simulink model "testing_model"  (R2024a)
settings: Solver=FixedStepAuto  StartTime=0.0  StopTime=60  FixedStep=Ts  RelTol=1e-3
values from neighbouring files (symbols this model uses):
  telescope0 = 0    [enviroment_setup.m]
  thetaList0 = [0, 0,-pi/8, 0, 0]'    [enviroment_setup.m]
  Ts = 0.001    [enviroment_setup.m]
libraries: TcSimInterface x2, sldrtlib x1
(part 2 of 2)

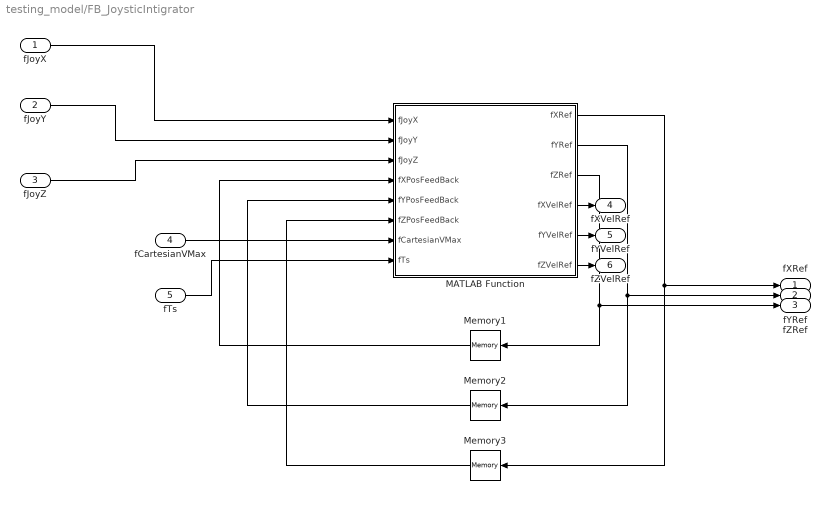
== system testing_model/FB_JoysticIntigrator ==
  fJoyX : Inport
  fJoyY : Inport  Port=2
  fJoyZ : Inport  Port=3
  fCartesianVMax : Inport  Port=4
  fTs : Inport  Port=5
  MATLAB Function : MATLAB Function  TreatAsAtomicUnit=on
  Memory1 : Memory
  Memory2 : Memory
  Memory3 : Memory
  fXRef : Outport
  fYRef : Outport  Port=2
  fZRef : Outport  Port=3
  fXVelRef : Outport  Port=4
  fYVelRef : Outport  Port=5
  fZVelRef : Outport  Port=6
  wires:
  Memory2/1 -> MATLAB Function/5(fYPosFeedBack)
  fJoyY/1 -> MATLAB Function/2(fJoyY)
  MATLAB Function/1(fXRef) -> fXRef/1, Memory3/1
  Memory1/1 -> MATLAB Function/4(fXPosFeedBack)
  MATLAB Function/2(fYRef) -> fYRef/1, Memory2/1
  fCartesianVMax/1 -> MATLAB Function/7(fCartesianVMax)
  Memory3/1 -> MATLAB Function/6(fZPosFeedBack)
  MATLAB Function/3(fZRef) -> fZRef/1, Memory1/1
  MATLAB Function/6(fZVelRef) -> fZVelRef/1
  MATLAB Function/4(fXVelRef) -> fXVelRef/1
  MATLAB Function/5(fYVelRef) -> fYVelRef/1
  fTs/1 -> MATLAB Function/8(fTs)
  fJoyX/1 -> MATLAB Function/1(fJoyX)
  fJoyZ/1 -> MATLAB Function/3(fJoyZ)

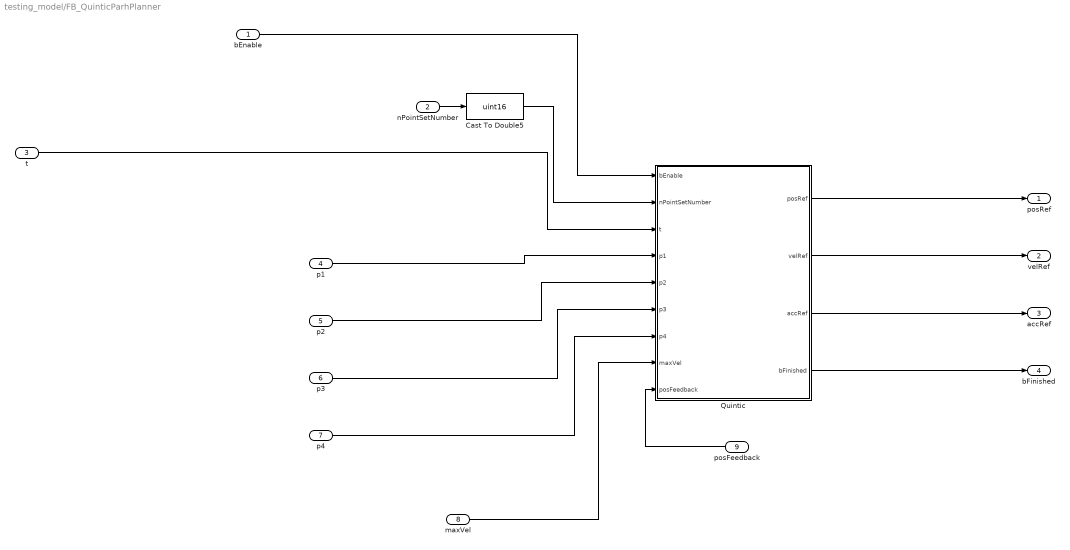
== system testing_model/FB_QuinticParhPlanner ==
  bEnable : Inport
  nPointSetNumber : Inport  Port=2
  t : Inport  Port=3
  p1 : Inport  Port=4
  p2 : Inport  Port=5
  p3 : Inport  Port=6
  p4 : Inport  Port=7
  maxVel : Inport  Port=8
  posFeedback : Inport  Port=9
  Cast To Double5 : DataTypeConversion  OutDataTypeStr=uint16  SaturateOnIntegerOverflow=off  RndMeth=Floor
  Quintic : MATLAB Function  TreatAsAtomicUnit=on
  posRef : Outport
  velRef : Outport  Port=2
  accRef : Outport  Port=3
  bFinished : Outport  Port=4
  wires:
  t/1 -> Quintic/3(t)
  p2/1 -> Quintic/5(p2)
  bEnable/1 -> Quintic/1(bEnable)
  maxVel/1 -> Quintic/8(maxVel)
  Quintic/4(bFinished) -> bFinished/1
  Quintic/2(velRef) -> velRef/1
  Quintic/1(posRef) -> posRef/1
  Quintic/3(accRef) -> accRef/1
  p1/1 -> Quintic/4(p1)
  p3/1 -> Quintic/6(p3)
  p4/1 -> Quintic/7(p4)
  posFeedback/1 -> Quintic/9(posFeedback)
  nPointSetNumber/1 -> Cast To Double5/1
  Cast To Double5/1 -> Quintic/2(nPointSetNumber)

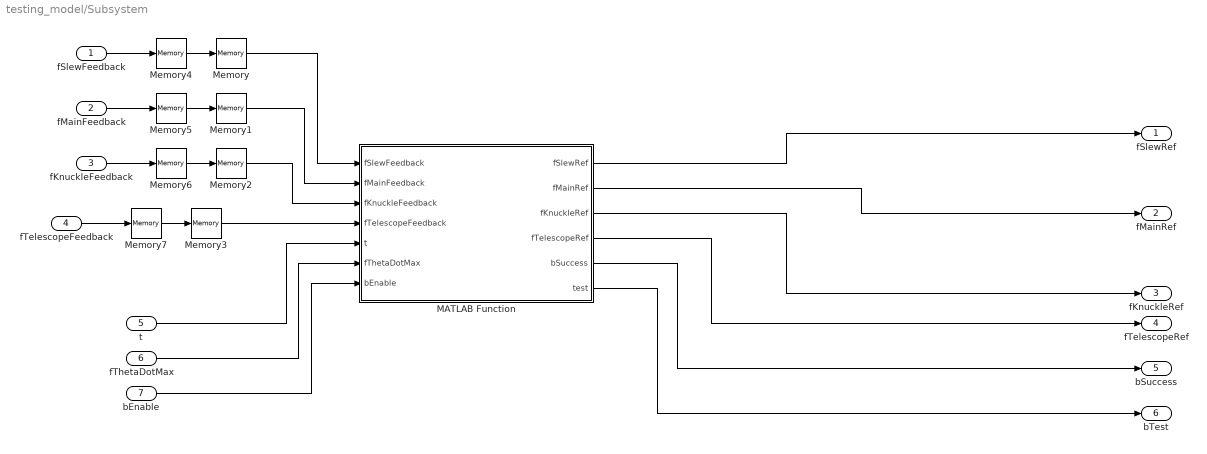
== system testing_model/Subsystem ==
  fSlewFeedback : Inport
  fMainFeedback : Inport  Port=2
  fKnuckleFeedback : Inport  Port=3
  fTelescopeFeedback : Inport  Port=4
  t : Inport  Port=5
  fThetaDotMax : Inport  Port=6
  bEnable : Inport  Port=7
  MATLAB Function : MATLAB Function  TreatAsAtomicUnit=on
  Memory : Memory  InitialCondition=thetaList0(1)
  Memory1 : Memory  InitialCondition=thetaList0(2)
  Memory2 : Memory  InitialCondition=thetaList0(3)
  Memory3 : Memory  InitialCondition=telescope0
  Memory4 : Memory  InitialCondition=thetaList0(1)
  Memory5 : Memory  InitialCondition=thetaList0(2)
  Memory6 : Memory  InitialCondition=thetaList0(3)
  Memory7 : Memory  InitialCondition=telescope0
  fSlewRef : Outport
  fMainRef : Outport  Port=2
  fKnuckleRef : Outport  Port=3
  fTelescopeRef : Outport  Port=4
  bSuccess : Outport  Port=5
  bTest : Outport  Port=6
  wires:
  MATLAB Function/4(fTelescopeRef) -> fTelescopeRef/1
  MATLAB Function/2(fMainRef) -> fMainRef/1
  fMainFeedback/1 -> Memory5/1
  fSlewFeedback/1 -> Memory4/1
  fKnuckleFeedback/1 -> Memory6/1
  MATLAB Function/5(bSuccess) -> bSuccess/1
  t/1 -> MATLAB Function/5(t)
  MATLAB Function/1(fSlewRef) -> fSlewRef/1
  MATLAB Function/3(fKnuckleRef) -> fKnuckleRef/1
  fThetaDotMax/1 -> MATLAB Function/6(fThetaDotMax)
  bEnable/1 -> MATLAB Function/7(bEnable)
  fTelescopeFeedback/1 -> Memory7/1
  Memory/1 -> MATLAB Function/1(fSlewFeedback)
  Memory1/1 -> MATLAB Function/2(fMainFeedback)
  Memory2/1 -> MATLAB Function/3(fKnuckleFeedback)
  Memory3/1 -> MATLAB Function/4(fTelescopeFeedback)
  Memory7/1 -> Memory3/1
  Memory4/1 -> Memory/1
  Memory5/1 -> Memory1/1
  Memory6/1 -> Memory2/1
  MATLAB Function/6(test) -> bTest/1

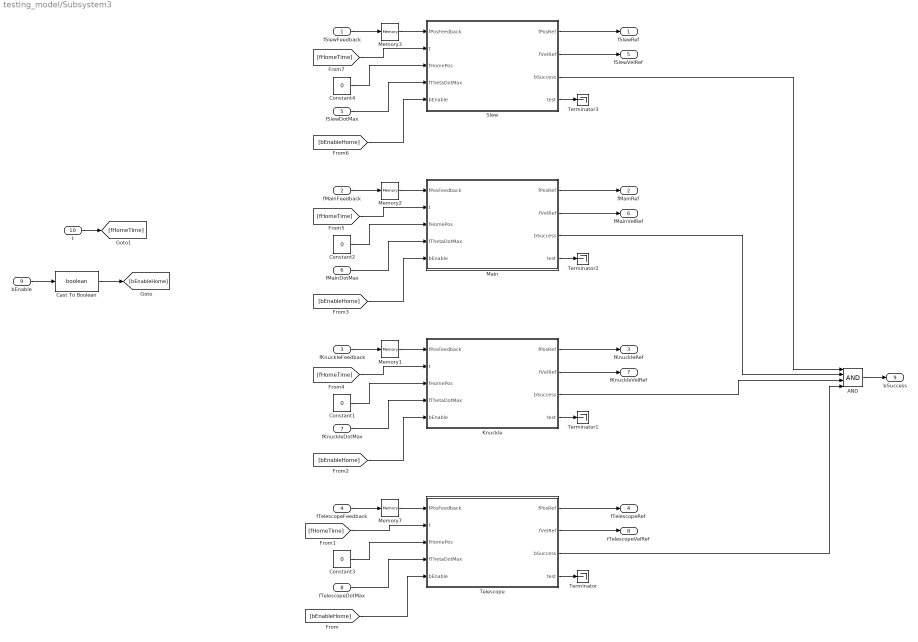
== system testing_model/Subsystem3 ==
  fSlewFeedback : Inport
  fMainFeedback : Inport  Port=2
  fKnuckleFeedback : Inport  Port=3
  fTelescopeFeedback : Inport  Port=4
  fSlewDotMax : Inport  Port=5
  fMainDotMax : Inport  Port=6
  fKnuckleDotMax : Inport  Port=7
  fTelescopeDotMax : Inport  Port=8
  bEnable : Inport  Port=9
  t : Inport  Port=10
  AND : Logic  Inputs=4  IconShape=distinctive  AllPortsSameDT=off  OutDataTypeStr=boolean
  Cast To Boolean : DataTypeConversion  OutDataTypeStr=boolean  SaturateOnIntegerOverflow=off  RndMeth=Floor
  Constant{1..4} (4 alike) : Constant  Value=0
  Knuckle : MATLAB Function  TreatAsAtomicUnit=on
  Main : MATLAB Function  TreatAsAtomicUnit=on
  Memory1 : Memory  InitialCondition=thetaList0(3)
  Memory2 : Memory  InitialCondition=thetaList0(2)
  Memory3 : Memory  InitialCondition=thetaList0(2)
  Memory7 : Memory  InitialCondition=telescope0
  Slew : MATLAB Function  TreatAsAtomicUnit=on
  Telescope : MATLAB Function  TreatAsAtomicUnit=on
  Terminator{,1..3} (4 alike) : Terminator
  fSlewRef : Outport
  fMainRef : Outport  Port=2
  fKnuckleRef : Outport  Port=3
  fTelescopeRef : Outport  Port=4
  fSlewVelRef : Outport  Port=5
  fMainVelRef : Outport  Port=6
  fKnuckleVelRef : Outport  Port=7
  fTelescopeVelRef : Outport  Port=8
  bSuccess : Outport  Port=9
  wires:
  Telescope/1(fPosRef) -> fTelescopeRef/1
  Telescope/3(bSuccess) -> AND/4
  [fHomeTime] -> Telescope/2(t)
  fTelescopeDotMax/1 -> Telescope/4(fThetaDotMax)
  [bEnableHome] -> Telescope/5(bEnable)
  fTelescopeFeedback/1 -> Memory7/1
  Constant3/1 -> Telescope/3(fHomePos)
  Memory7/1 -> Telescope/1(fPosFeedback)
  Telescope/2(fVelRef) -> fTelescopeVelRef/1
  Telescope/4(test) -> Terminator/1
  Constant1/1 -> Knuckle/3(fHomePos)
  Knuckle/3(bSuccess) -> AND/3
  Knuckle/2(fVelRef) -> fKnuckleVelRef/1
  Memory1/1 -> Knuckle/1(fPosFeedback)
  Knuckle/4(test) -> Terminator1/1
  Knuckle/1(fPosRef) -> fKnuckleRef/1
  [bEnableHome] -> Knuckle/5(bEnable)
  fKnuckleDotMax/1 -> Knuckle/4(fThetaDotMax)
  [fHomeTime] -> Knuckle/2(t)
  fKnuckleFeedback/1 -> Memory1/1
  AND/1 -> bSuccess/1
  bEnable/1 -> Cast To Boolean/1
  t/1 -> [fHomeTime]
  Cast To Boolean/1 -> [bEnableHome]
  Main/3(bSuccess) -> AND/2
  fMainDotMax/1 -> Main/4(fThetaDotMax)
  Main/4(test) -> Terminator2/1
  fMainFeedback/1 -> Memory2/1
  Memory2/1 -> Main/1(fPosFeedback)
  Main/2(fVelRef) -> fMainVelRef/1
  [bEnableHome] -> Main/5(bEnable)
  Constant2/1 -> Main/3(fHomePos)
  Main/1(fPosRef) -> fMainRef/1
  [fHomeTime] -> Main/2(t)
  [bEnableHome] -> Slew/5(bEnable)
  Slew/2(fVelRef) -> fSlewVelRef/1
  Memory3/1 -> Slew/1(fPosFeedback)
  Slew/3(bSuccess) -> AND/1
  Slew/4(test) -> Terminator3/1
  [fHomeTime] -> Slew/2(t)
  Slew/1(fPosRef) -> fSlewRef/1
  fSlewFeedback/1 -> Memory3/1
  Constant4/1 -> Slew/3(fHomePos)
  fSlewDotMax/1 -> Slew/4(fThetaDotMax)

== matlab function testing_model/FB_JoysticIntigrator/MATLAB Function ==
  data: fJoyX input; fJoyY input; fJoyZ input; fXPosFeedBack input; fXRef output; fYRef output; fZRef output; fXVelRef output; fYVelRef output; fZVelRef output; fYPosFeedBack input; fZPosFeedBack input; fCartesianVMax input; fTs input
function [fXRef, fYRef, fZRef, fXVelRef, fYVelRef, fZVelRef]  = fcn(fJoyX, fJoyY, fJoyZ, fXPosFeedBack, fYPosFeedBack, fZPosFeedBack, fCartesianVMax, fTs)

fXVelRef = fCartesianVMax*fJoyX;
fYVelRef = fCartesianVMax*fJoyY;
fZVelRef = fCartesianVMax*fJoyZ;

fXRef = fXPosFeedBack + fXVelRef*fTs;
fYRef = fYPosFeedBack + fYVelRef*fTs; 
fZRef = fZPosFeedBack + fZVelRef*fTs;

== matlab function testing_model/MATLAB Function3 ==
  settings: updateMethod=DISCRETE
  data: p1 input; p2 input; p3 input; xyzOut output; xyzDotOut output; t_current input; bEnable input; MaxVel input; pointSetNumber input; pointSetFromMemory input; pointSetToMemory output; xyzFeedback input; xyzDotFeedback input; tFromMemory input; tToMemory output
function [xyzOut, xyzDotOut, pointSetToMemory, tToMemory] = CubicPlanner(p1, p2, p3, t_current, bEnable, MaxVel, pointSetNumber, pointSetFromMemory, xyzFeedback, xyzDotFeedback,tFromMemory)
xyzOut = zeros(3, 1);
xyzDotOut = zeros(3, 1);
bFirstCycle = false;
bNewPointSet = false;


persistent tToSubtract;
if isempty(tToSubtract)
    tToSubtract = 0.0;
end

persistent bEnableMemory;
if isempty(bEnableMemory)
    bEnableMemory = false;
end

persistent p1Memory;
if isempty(p1Memory)
    p1Memory = p1;
end
persistent p2Memory;
if isempty(p2Memory)
    p2Memory = p2;
end
persistent p3Memory;
if isempty(p3Memory)
    p3Memory = p3;
end


% Detect first cykle
if (bEnable == true) && (bEnableMemory == false)
    bFirstCycle = true;
end

% Detecet new pointset:
if (pointSetNumber) == (pointSetFromMemory + 1)
    bNewPointSet = true;
end


% Detect new pointset or enable pressed then subract time.
if bNewPointSet || bFirstCycle
    tToSubtract = t_current;
end
t_current = t_current - tToSubtract;

if ~bEnable
    xyzOut = xyzFeedback;
    xyzDotOut = zeros(3, 1);
    pointSetToMemory = pointSetFromMemory;
    tToMemory = t_current;
    bEnableMemory = bEnable;
    return;
end

% Write new points to memory if new point set is detected
if bNewPointSet
    p1Memory = p1;
    p2Memory = p2;
    p3Memory = p3;
end

% Position (xyz) and time vectors
%px = [4.55, 0, 2];
%py = [0.4, 3.5, 2];
%pz = [1.6,  1.9,  2];



px = [0, p1Memory(1,1), p2Memory(1,1), p3Memory(1, 1)];
py = [0, p1Memory(2,1), p2Memory(2,1), p3Memory(2, 1)];
pz = [0, p1Memory(3,1), p2Memory(3,1), p3Memory(3, 1)];



% Calculating time based on distance and max velocity
tTemp1 =  [px(1), px(1), py(1)] - [px(2), px(2), py(2)];
tTemp2 =  [px(2), px(2), py(2)] - [px(3), px(3), py(3)];
tTemp3 =  [px(3), px(3), py(3)] - [px(4), px(4), py(4)];
t1 = norm(tTemp1)/MaxVel;
t2 = norm(tTemp2)/MaxVel;
t3 = norm(tTemp3)/MaxVel;
t =  [0,  t1, (t1 + t2), (t1 + t2 + t3)];



if(t_current >= t(end))
    t_current = t(end);
end


%palpha = [0 0 0 0 pi/4 0 0];

pt = [px; py; pz]';

%v = 0.005;


vx = [0 MaxVel MaxVel 0];
vy = [0 MaxVel MaxVel 0];
vz = [0 MaxVel MaxVel 0];

if(t_current < t(2))
    idx = 1;
elseif(t_current < t(3))
    idx = 2;
elseif(t_current < t(4))
    idx = 3;
else
    idx = 3;
end


t0 = t(idx);

x0 = pt(idx,  1);
x1 = pt(idx+1,1);
y0 = pt(idx,  2);
y1 = pt(idx+1,2);
z0 = pt(idx,  3);
z1 = pt(idx+1,3);

v0_x = vx(idx);
v1_x = vx(idx+1);

v0_y = vy(idx);
v1_y = vy(idx+1);

v0_z = vz(idx);
v1_z = vz(idx+1);

%alpha0 = palpha(idx);
%alpha1 = palpha(idx+1);

t1 = t(idx+1);
if(t_current < t(length(px)))
    [x, x_t] = CubicRT(t0, t1, t_current, x0, x1, v0_x, v1_x);
    [y, y_t] = CubicRT(t0, t1, t_current, y0, y1, v0_y, v1_y);
    [z, z_t] = CubicRT(t0, t1, t_current, z0, z1, v0_z, v1_z);
    %[alpha, alpha_t] = QuinticRT(t0, t1, t_current, alpha0, alpha1, 0, 0.001);
else
    x = px(length(px));
    y = py(length(py));
    z = pz(length(pz));
    x_t = 0;
    y_t = 0;
    z_t = 0;
    %alpha_t = 0;
end

xyzOut(1, 1) = x;
xyzOut(2, 1) = y;
xyzOut(3, 1) = z;

xyzDotOut(1, 1) = x_t;
xyzDotOut(2, 1) = y_t;
xyzDotOut(3, 1) = z_t;


% Write to memory
pointSetToMemory = pointSetNumber;
tToMemory = t_current;
bEnableMemory = bEnable;
end

== matlab function testing_model/FB_QuinticParhPlanner/Quintic ==
  data: bEnable input; nPointSetNumber input; posRef output; t input; velRef output; accRef output; p1 input; p2 input; p3 input; p4 input; maxVel input; bFinished output; posFeedback input
function [posRef, velRef, accRef, bFinished] = QuinticGenerator( ...
    bEnable, nPointSetNumber, t, p1, p2, p3, p4, maxVel, posFeedback )
% QUINTICGENERATOR
%   Generates piecewise polynomial references (pos/vel/acc) for up to 4 segments.
%   Re-computes polynomials only when nPointSetNumber increments (signaling
%   a new waypoint set), and only if bEnable == true.
%
%   If bEnable is false, outputs a stationary reference at posFeedback.

    %%% PERSISTENT VARIABLES %%%%%%%%%%%%%%%%%%%%%%%%%%%%%%%%%%%%%%%%%%%%%
    persistent bEnableMemory                % Remember last enable state
    persistent pointSetNumberMemory         % Remember last waypoint-set counter
    
    persistent p1Memory p2Memory p3Memory p4Memory
    persistent timeSlotsMemory
    persistent coeffXMemory coeffYMemory coeffZMemory
    persistent posRefMemory velRefMemory accRefMemory
    persistent t0Memory                    % Local start time offset
    
    % Initialize persistent variables if empty
    if isempty(bEnableMemory),       bEnableMemory       = false;      end
    if isempty(pointSetNumberMemory),pointSetNumberMemory= uint16(0);  end
    
    if isempty(p1Memory),           p1Memory            = zeros(3,1); end
    if isempty(p2Memory),           p2Memory            = zeros(3,1); end
    if isempty(p3Memory),           p3Memory            = zeros(3,1); end
    if isempty(p4Memory),           p4Memory            = zeros(3,1); end
    
    if isempty(timeSlotsMemory),     timeSlotsMemory     = [0 1 2 3 4];end
    if isempty(coeffXMemory),        coeffXMemory        = zeros(18,1);end
    if isempty(coeffYMemory),        coeffYMemory        = zeros(18,1);end
    if isempty(coeffZMemory),        coeffZMemory        = zeros(18,1);end
    
    if isempty(posRefMemory),        posRefMemory        = posFeedback; end
    if isempty(velRefMemory),        velRefMemory        = zeros(3,1); end
    if isempty(accRefMemory),        accRefMemory        = zeros(3,1); end
    
    if isempty(t0Memory),           t0Memory            = 0;          end

    %%% DEFAULT OUTPUTS (if bEnable == false) %%%%%%%%%%%%%%%%%%%%%%%%%%%%
    %   Stationary reference at the current feedback position
    posRef    = posFeedback;   
    velRef    = zeros(3,1);
    accRef    = zeros(3,1);
    bFinished = true;  % Not actively running any trajectory
    bFirsCykle = false;
    %----------------------------------------------------------------------
    % 1) CHECK IF DISABLED => Return a stationary reference immediately
    %----------------------------------------------------------------------
    if ~bEnable
        % Make sure to remember we are now disabled
        bEnableMemory = false;
        return;
    end

    %----------------------------------------------------------------------
    % 2) IF WE GET HERE => bEnable == true
    %    We want to see if we just transitioned from false->true
    %----------------------------------------------------------------------
    if bEnable && ~bEnableMemory
        % Rising edge of bEnable => reset local start time
        %t0Memory = t;
        bFirsCykle = true;
    end
    
    % Update bEnableMemory to reflect the current state
    bEnableMemory = true;

    %----------------------------------------------------------------------
    % 3) Check if nPointSetNumber has incremented => new waypoints
    %----------------------------------------------------------------------
    if nPointSetNumber > pointSetNumberMemory
        bNewPointSet = true;
        pointSetNumberMemory = nPointSetNumber;
    else
        bNewPointSet = false;
    end
        
    %reset local start time
    if bFirsCykle | bNewPointSet
        t0Memory = t;
    end


    %----------------------------------------------------------------------
    % 4) If new points, compute new polynomials
    %    We only do this if we are enabled (which we are) 
    %----------------------------------------------------------------------
    if bNewPointSet
        % Save new waypoints
        p1Memory = p1;
        p2Memory = p2;
        p3Memory = p3;
        p4Memory = p4;
        
        % We can choose velocity/accel for start from the *old* memory 
        % or from zero. Example: from memory
        v0x = velRefMemory(1);  a0x = accRefMemory(1);
        v0y = velRefMemory(2);  a0y = accRefMemory(2);
        v0z = velRefMemory(3);  a0z = accRefMemory(3);

        % Build vectors of 5 points in each dimension
        % Start from the current feedback (or last posRefMemory),
        % but commonly we use posFeedback for a fresh start.
        xPoints = [posFeedback(1), p1(1), p2(1), p3(1), p4(1)];
        yPoints = [posFeedback(2), p1(2), p2(2), p3(2), p4(2)];
        zPoints = [posFeedback(3), p1(3), p2(3), p3(3), p4(3)];

        % Time computations
        maxVel3D = maxVel / sqrt(3);  % if you want sqrt(vx^2 + vy^2 + vz^2) = maxVel
        dTemp1 = [xPoints(1), yPoints(1), zPoints(1)] - [xPoints(2), yPoints(2), zPoints(2)];
        dTemp2 = [xPoints(2), yPoints(2), zPoints(2)] - [xPoints(3), yPoints(3), zPoints(3)];
        dTemp3 = [xPoints(3), yPoints(3), zPoints(3)] - [xPoints(4), yPoints(4), zPoints(4)];
        dTemp4 = [xPoints(4), yPoints(4), zPoints(4)] - [xPoints(5), yPoints(5), zPoints(5)];

        t1 = norm(dTemp1) / maxVel3D;
        t2 = norm(dTemp2) / maxVel3D;
        t3 = norm(dTemp3) / maxVel3D;
        t4 = norm(dTemp4) / maxVel3D;
        
        timeSlots = [0, t1, t1 + t2, t1 + t2 + t3, t1 + t2 + t3 + t4];
        timeSlotsMemory = timeSlots;

        % Compute polynomials (Quintic)
        coeffX = Quintic(timeSlots, xPoints, v0x, a0x);
        coeffY = Quintic(timeSlots, yPoints, v0y, a0y);
        coeffZ = Quintic(timeSlots, zPoints, v0z, a0z);
        
        coeffXMemory = coeffX;
        coeffYMemory = coeffY;
        coeffZMemory = coeffZ;
    end

    %----------------------------------------------------------------------
    % 5) Evaluate polynomials at local time => tLocal = t - t0Memory
    %----------------------------------------------------------------------
    tLocal = t - t0Memory;

    % If local time is beyond the final timeSlot => clamp & declare finished
    timeSlots = timeSlotsMemory;
    if tLocal >= timeSlots(end)
        tLocal = timeSlots(end);
        bFinished = true;
    else
        bFinished = false;
    end

    % Retrieve precomputed coefficients
    coeffX = coeffXMemory;
    coeffY = coeffYMemory;
    coeffZ = coeffZMemory;

    % Decide which segment to evaluate
    if tLocal < timeSlots(2)
        % Segment 1 (4th order)
        posRef = [F4(tLocal)*coeffX(1:5);
                  F4(tLocal)*coeffY(1:5);
                  F4(tLocal)*coeffZ(1:5)];

        velRef = [F4Dot(tLocal)*coeffX(1:5);
                  F4Dot(tLocal)*coeffY(1:5);
                  F4Dot(tLocal)*coeffZ(1:5)];

        accRef = [F4DotDot(tLocal)*coeffX(1:5);
                  F4DotDot(tLocal)*coeffY(1:5);
                  F4DotDot(tLocal)*coeffZ(1:5)];

    elseif tLocal < timeSlots(3)
        % Segment 2 (3rd order)
        posRef = [F3(tLocal)*coeffX(6:9);
                  F3(tLocal)*coeffY(6:9);
                  F3(tLocal)*coeffZ(6:9)];

        velRef = [F3Dot(tLocal)*coeffX(6:9);
                  F3Dot(tLocal)*coeffY(6:9);
                  F3Dot(tLocal)*coeffZ(6:9)];

        accRef = [F3DotDot(tLocal)*coeffX(6:9);
                  F3DotDot(tLocal)*coeffY(6:9);
                  F3DotDot(tLocal)*coeffZ(6:9)];

    elseif tLocal < timeSlots(4)
        % Segment 3 (3rd order)
        posRef = [F3(tLocal)*coeffX(10:13);
                  F3(tLocal)*coeffY(10:13);
                  F3(tLocal)*coeffZ(10:13)];

        velRef = [F3Dot(tLocal)*coeffX(10:13);
                  F3Dot(tLocal)*coeffY(10:13);
                  F3Dot(tLocal)*coeffZ(10:13)];

        accRef = [F3DotDot(tLocal)*coeffX(10:13);
                  F3DotDot(tLocal)*coeffY(10:13);
                  F3DotDot(tLocal)*coeffZ(10:13)];
              
    else
        % Segment 4 (4th order)
        posRef = [F4(tLocal)*coeffX(14:18);
                  F4(tLocal)*coeffY(14:18);
                  F4(tLocal)*coeffZ(14:18)];

        velRef = [F4Dot(tLocal)*coeffX(14:18);
                  F4Dot(tLocal)*coeffY(14:18);
                  F4Dot(tLocal)*coeffZ(14:18)];

        accRef = [F4DotDot(tLocal)*coeffX(14:18);
                  F4DotDot(tLocal)*coeffY(14:18);
                  F4DotDot(tLocal)*coeffZ(14:18)];
    end

    %----------------------------------------------------------------------
    % 6) Save references to memory for next cycle
    %----------------------------------------------------------------------
    posRefMemory = posRef;
    velRefMemory = velRef;
    accRefMemory = accRef;

end

== matlab function testing_model/Subsystem/MATLAB Function ==
  settings: updateMethod=DISCRETE
  data: fSlewFeedback input; fSlewRef output; fMainRef output; fKnuckleRef output; fTelescopeRef output; fMainFeedback input; fKnuckleFeedback input; fTelescopeFeedback input; t input; bSuccess output; fThetaDotMax input; bEnable input; test output
function [fSlewRef, fMainRef, fKnuckleRef, fTelescopeRef, bSuccess, test] = ...
                    goHome(fSlewFeedback, ...
                    fMainFeedback, ...
                    fKnuckleFeedback, ...
                    fTelescopeFeedback, ...
                    t,...
                    fThetaDotMax, ...
                    bEnable)
bSuccess = false;


%fSlewRef = 0;
%fMainRef = 0;
%fKnuckleRef = 0;
%fTelescopeRef = 0;

slewHomeTheta = 0.0;
mainHomeTheta = 0.0;
knuckleHomeTheta = 0.0;
telescopeHomeTheta = 2.0;


[fSlewRef, ~, bSlewDone, ~] = cosinePositionGenerator(fSlewFeedback, slewHomeTheta, fThetaDotMax, t, bEnable);
[fMainRef, ~, bMainDone, ~] = cosinePositionGenerator(fMainFeedback, mainHomeTheta, fThetaDotMax, t, bEnable);
[fKnuckleRef, ~, bKnuckleDone, ~] = cosinePositionGenerator(fKnuckleFeedback, knuckleHomeTheta, fThetaDotMax, t, bEnable);

[fTelescopeRef, ~, bTelescopeDone, test] = cosinePositionGenerator(fTelescopeFeedback, telescopeHomeTheta, fThetaDotMax, t, bEnable);

if (bSlewDone & bMainDone & bKnuckleDone & bTelescopeDone)
    bSuccess = true;
end



end

== matlab function testing_model/Subsystem3/Knuckle ==
  settings: updateMethod=DISCRETE
  data: fPosRef output; fVelRef output; fPosFeedback input; t input; fHomePos input; bSuccess output; fThetaDotMax input; bEnable input; test output
function [fPosRef, fVelRef, bSuccess, test] = goHomeKnuckle(fPosFeedback, ...
    t,...
    fHomePos,...
    fThetaDotMax, ...
    bEnable)

bSuccess = false;
fPosRef = 0.0;
fVelRef = 0.0;
test = false;




[fPosRef, fVelRef, bSuccess, test] = cosinePositionGenerator(fPosFeedback, fHomePos, fThetaDotMax, t, bEnable);



end

== matlab function testing_model/Subsystem3/Main ==
  settings: updateMethod=DISCRETE
  data: fPosRef output; fVelRef output; fPosFeedback input; t input; fHomePos input; bSuccess output; fThetaDotMax input; bEnable input; test output
function [fPosRef, fVelRef, bSuccess, test] = goHomeMain(fPosFeedback, ...
    t,...
    fHomePos,...
    fThetaDotMax, ...
    bEnable)

bSuccess = false;
fPosRef = 0.0;
fVelRef = 0.0;
test = false;




[fPosRef, fVelRef, bSuccess, test] = cosinePositionGenerator(fPosFeedback, fHomePos, fThetaDotMax, t, bEnable);



end

== matlab function testing_model/Subsystem3/Slew ==
  settings: updateMethod=DISCRETE
  data: fPosRef output; fVelRef output; fPosFeedback input; t input; fHomePos input; bSuccess output; fThetaDotMax input; bEnable input; test output
function [fPosRef, fVelRef, bSuccess, test] = goHomeSlew(fPosFeedback, ...
    t,...
    fHomePos,...
    fThetaDotMax, ...
    bEnable)

bSuccess = false;
fPosRef = 0.0;
fVelRef = 0.0;
test = false;




[fPosRef, fVelRef, bSuccess, test] = cosinePositionGenerator(fPosFeedback, fHomePos, fThetaDotMax, t, bEnable);



end

== matlab function testing_model/Subsystem3/Telescope ==
  settings: updateMethod=DISCRETE
  data: fPosRef output; fVelRef output; fPosFeedback input; t input; fHomePos input; bSuccess output; fThetaDotMax input; bEnable input; test output
function [fPosRef, fVelRef, bSuccess, test] = goHomeTelescope(fPosFeedback, ...
    t,...
    fHomePos,...
    fThetaDotMax, ...
    bEnable)

bSuccess = false;
fPosRef = 0.0;
fVelRef = 0.0;
test = false;


[fPosRef, fVelRef, bSuccess, test] = cosinePositionGenerator(fPosFeedback, fHomePos, fThetaDotMax, t, bEnable);



end
